simulink model "Pendulum"  (R2021a)
settings: Solver=VariableStepAuto  StartTime=0.0  StopTime=80.0  RelTol=1e-3
undefined symbols (not defined in the file): c, d, g, J, L, m
libraries: simulink_extras x2, fuzblock x1
settings Model: SimulationMode=rapid-accelerator  Creator=ejbejaranos  LastModifiedBy=ejbejaranos

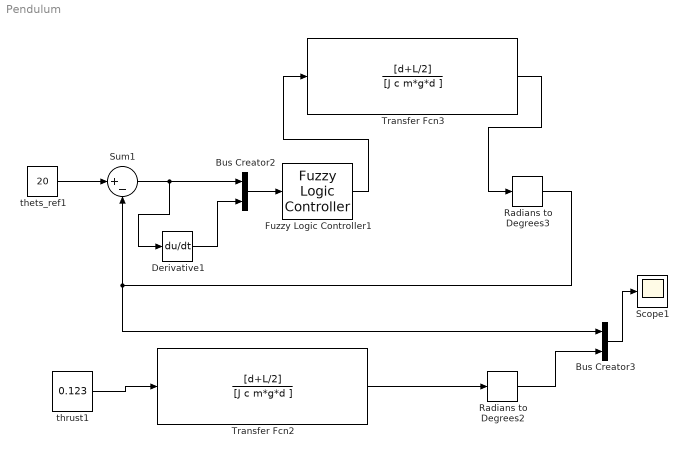
== system Pendulum ==
  Bus Creator2 : BusCreator  Inputs=2
  Bus Creator3 : BusCreator  Inputs=2
  Derivative1 : Derivative
  Fuzzy Logic Controller1 : fuzblock/Fuzzy Logic  Controller  FIS=mandami_output5mf  OutputSampleNumber=101  DataType=double  FuzzifiedInputs=off  RuleFiringStrengths=off  RuleOutputs=off  AggregatedOutputs=off  SimulateUsing=Interpreted execution  OutOfRangeInputValueMessage=warning  NoRuleFiredMessage=warning  EmptyOutputFuzzySetMessage=warning
  Radians to Degrees2 : simulink_extras/Transformations/Radians to Degrees
  Radians to Degrees3 : simulink_extras/Transformations/Radians to Degrees
  Scope1 : Scope
  Sum1 : Sum  Inputs=|+-
  Transfer Fcn2 : TransferFcn  Numerator=[d+L/2]  Denominator=[J c m*g*d ]
  Transfer Fcn3 : TransferFcn  Numerator=[d+L/2]  Denominator=[J c m*g*d ]
  thets_ref1 : Constant  Value=20
  thrust1 : Constant  Value=0.123
  wires:
  Transfer Fcn3/1 -> Radians to Degrees3/1
  Fuzzy Logic Controller1/1 -> Transfer Fcn3/1
  Bus Creator2/1 -> Fuzzy Logic Controller1/1
  Derivative1/1 -> Bus Creator2/2
  Sum1/1 -> Derivative1/1, Bus Creator2/1
  thets_ref1/1 -> Sum1/1
  Bus Creator3/1 -> Scope1/1
  Radians to Degrees3/1 -> Bus Creator3/1, Sum1/2
  thrust1/1 -> Transfer Fcn2/1
  Transfer Fcn2/1 -> Radians to Degrees2/1
  Radians to Degrees2/1 -> Bus Creator3/2
